simulink model "Ecm_2RC_battery"  (R2022a)
settings: Solver=FixedStepAuto  StartTime=0.0  StopTime=3600  FixedStep=0.1  RelTol=1e-3
values from neighbouring files (symbols this model uses):
  T_init = 293.15    [cell_data.mat]
libraries: fl_lib x1074, LiBatteryElements_lib x540, nesl_utility x102
(part 2 of 18)

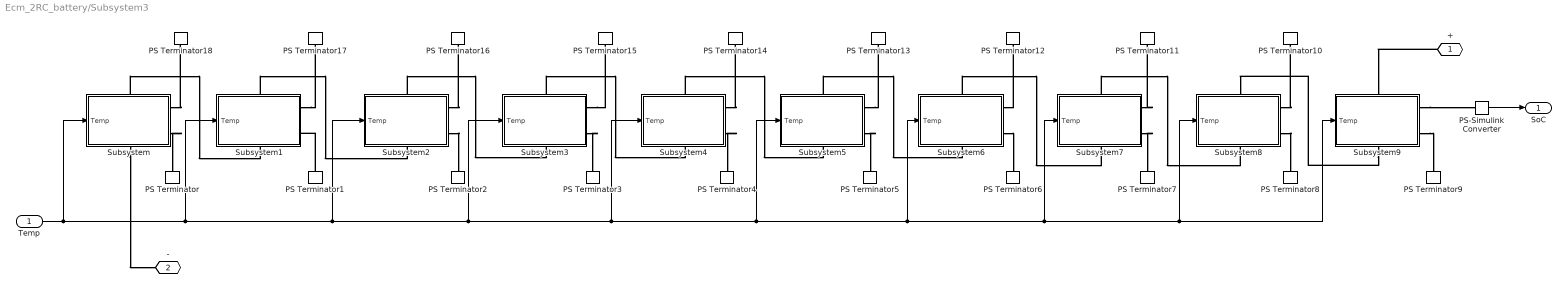
== system Ecm_2RC_battery/Subsystem3 ==
  Temp : Inport
  PS Terminator{,1..18} (19 alike) : fl_lib/Physical Signals/Sinks/PS Terminator
      settings: SourceProductBaseCode=PW,SS,VE
  PS-Simulink Converter : nesl_utility/PS-Simulink Converter  PhysicalDomain=network_engine_domain  SubClassName=ps_output  LeftPortType=input  RightPortType=output  PseudoPeriodic=off  Frequencies=[]  VectorFormat=inherit  Unit=inherit  AffineConversion=off
      settings: SourceProductBaseCode=SS,PW,VE
  Subsystem : Subsystem
      settings: PortSchema="{\"entries\":[{\"content\":{\"sides\":[{\"content\":{\"connectorIds\":[\"In1\"]},\"type\":\"ConnectorPlacement.EquallySpacedRectSide\",\"uuid\":\"c40d362d-5d22-4f8a-8be9-1546116d818f\"},{\"content\":{\"connectorIds\":[\"RConn1\",\"RConn2\"],\"side\":\"RIGHT\"},\"type\":\"ConnectorPlacement.EquallySpacedRectSide\",\"uuid\":\"b280b04f-a99a-4e6d-85c5-70766288d403\"},{\"content\":{\"connectorIds\":[\"LConn1\"],\"side\":\"TOP\"},\"type\":\"ConnectorPlacement.EquallySpacedRectSide\",\"uuid\":\"c08bcee5-d382-416b-973d-9a8915fb752a\"},{\"content\":{\"connectorIds\":[\"RConn3\"],\"side\":\"BOTTOM\"},\"type\":\"ConnectorPlacement.EquallySpacedRectSide\",\"uuid\":\"7b01a887-c5d2-42f0-ba08-9cc04bc53540\"}]},\"type\":\"ConnectorPlacement.EquallySpacedConnector\",\"uuid\":\"7a443456-32e2-4b79-b23a-7f1f6189d6a8\"}],\"packageUris\":[\"http://schema.mathworks.com/mf0/Connector/R2020b\"],\"version\":\"1.0\"}"
  Subsystem1 : Subsystem
      settings: PortSchema="{\"entries\":[{\"content\":{\"sides\":[{\"content\":{\"connectorIds\":[\"In1\"]},\"type\":\"ConnectorPlacement.EquallySpacedRectSide\",\"uuid\":\"c40d362d-5d22-4f8a-8be9-1546116d818f\"},{\"content\":{\"connectorIds\":[\"RConn1\",\"RConn2\"],\"side\":\"RIGHT\"},\"type\":\"ConnectorPlacement.EquallySpacedRectSide\",\"uuid\":\"b280b04f-a99a-4e6d-85c5-70766288d403\"},{\"content\":{\"connectorIds\":[\"LConn1\"],\"side\":\"TOP\"},\"type\":\"ConnectorPlacement.EquallySpacedRectSide\",\"uuid\":\"c08bcee5-d382-416b-973d-9a8915fb752a\"},{\"content\":{\"connectorIds\":[\"RConn3\"],\"side\":\"BOTTOM\"},\"type\":\"ConnectorPlacement.EquallySpacedRectSide\",\"uuid\":\"7b01a887-c5d2-42f0-ba08-9cc04bc53540\"}]},\"type\":\"ConnectorPlacement.EquallySpacedConnector\",\"uuid\":\"7a443456-32e2-4b79-b23a-7f1f6189d6a8\"}],\"packageUris\":[\"http://schema.mathworks.com/mf0/Connector/R2020b\"],\"version\":\"1.0\"}"
  Subsystem2 : Subsystem
      settings: PortSchema="{\"entries\":[{\"content\":{\"sides\":[{\"content\":{\"connectorIds\":[\"In1\"]},\"type\":\"ConnectorPlacement.EquallySpacedRectSide\",\"uuid\":\"c40d362d-5d22-4f8a-8be9-1546116d818f\"},{\"content\":{\"connectorIds\":[\"RConn1\",\"RConn2\"],\"side\":\"RIGHT\"},\"type\":\"ConnectorPlacement.EquallySpacedRectSide\",\"uuid\":\"b280b04f-a99a-4e6d-85c5-70766288d403\"},{\"content\":{\"connectorIds\":[\"LConn1\"],\"side\":\"TOP\"},\"type\":\"ConnectorPlacement.EquallySpacedRectSide\",\"uuid\":\"c08bcee5-d382-416b-973d-9a8915fb752a\"},{\"content\":{\"connectorIds\":[\"RConn3\"],\"side\":\"BOTTOM\"},\"type\":\"ConnectorPlacement.EquallySpacedRectSide\",\"uuid\":\"7b01a887-c5d2-42f0-ba08-9cc04bc53540\"}]},\"type\":\"ConnectorPlacement.EquallySpacedConnector\",\"uuid\":\"7a443456-32e2-4b79-b23a-7f1f6189d6a8\"}],\"packageUris\":[\"http://schema.mathworks.com/mf0/Connector/R2020b\"],\"version\":\"1.0\"}"
  Subsystem3 : Subsystem
      settings: PortSchema="{\"entries\":[{\"content\":{\"sides\":[{\"content\":{\"connectorIds\":[\"In1\"]},\"type\":\"ConnectorPlacement.EquallySpacedRectSide\",\"uuid\":\"c40d362d-5d22-4f8a-8be9-1546116d818f\"},{\"content\":{\"connectorIds\":[\"RConn1\",\"RConn2\"],\"side\":\"RIGHT\"},\"type\":\"ConnectorPlacement.EquallySpacedRectSide\",\"uuid\":\"b280b04f-a99a-4e6d-85c5-70766288d403\"},{\"content\":{\"connectorIds\":[\"LConn1\"],\"side\":\"TOP\"},\"type\":\"ConnectorPlacement.EquallySpacedRectSide\",\"uuid\":\"c08bcee5-d382-416b-973d-9a8915fb752a\"},{\"content\":{\"connectorIds\":[\"RConn3\"],\"side\":\"BOTTOM\"},\"type\":\"ConnectorPlacement.EquallySpacedRectSide\",\"uuid\":\"7b01a887-c5d2-42f0-ba08-9cc04bc53540\"}]},\"type\":\"ConnectorPlacement.EquallySpacedConnector\",\"uuid\":\"7a443456-32e2-4b79-b23a-7f1f6189d6a8\"}],\"packageUris\":[\"http://schema.mathworks.com/mf0/Connector/R2020b\"],\"version\":\"1.0\"}"
  Subsystem4 : Subsystem
      settings: PortSchema="{\"entries\":[{\"content\":{\"sides\":[{\"content\":{\"connectorIds\":[\"In1\"]},\"type\":\"ConnectorPlacement.EquallySpacedRectSide\",\"uuid\":\"c40d362d-5d22-4f8a-8be9-1546116d818f\"},{\"content\":{\"connectorIds\":[\"RConn1\",\"RConn2\"],\"side\":\"RIGHT\"},\"type\":\"ConnectorPlacement.EquallySpacedRectSide\",\"uuid\":\"b280b04f-a99a-4e6d-85c5-70766288d403\"},{\"content\":{\"connectorIds\":[\"LConn1\"],\"side\":\"TOP\"},\"type\":\"ConnectorPlacement.EquallySpacedRectSide\",\"uuid\":\"c08bcee5-d382-416b-973d-9a8915fb752a\"},{\"content\":{\"connectorIds\":[\"RConn3\"],\"side\":\"BOTTOM\"},\"type\":\"ConnectorPlacement.EquallySpacedRectSide\",\"uuid\":\"7b01a887-c5d2-42f0-ba08-9cc04bc53540\"}]},\"type\":\"ConnectorPlacement.EquallySpacedConnector\",\"uuid\":\"7a443456-32e2-4b79-b23a-7f1f6189d6a8\"}],\"packageUris\":[\"http://schema.mathworks.com/mf0/Connector/R2020b\"],\"version\":\"1.0\"}"
  Subsystem5 : Subsystem
      settings: PortSchema="{\"entries\":[{\"content\":{\"sides\":[{\"content\":{\"connectorIds\":[\"In1\"]},\"type\":\"ConnectorPlacement.EquallySpacedRectSide\",\"uuid\":\"c40d362d-5d22-4f8a-8be9-1546116d818f\"},{\"content\":{\"connectorIds\":[\"RConn1\",\"RConn2\"],\"side\":\"RIGHT\"},\"type\":\"ConnectorPlacement.EquallySpacedRectSide\",\"uuid\":\"b280b04f-a99a-4e6d-85c5-70766288d403\"},{\"content\":{\"connectorIds\":[\"LConn1\"],\"side\":\"TOP\"},\"type\":\"ConnectorPlacement.EquallySpacedRectSide\",\"uuid\":\"c08bcee5-d382-416b-973d-9a8915fb752a\"},{\"content\":{\"connectorIds\":[\"RConn3\"],\"side\":\"BOTTOM\"},\"type\":\"ConnectorPlacement.EquallySpacedRectSide\",\"uuid\":\"7b01a887-c5d2-42f0-ba08-9cc04bc53540\"}]},\"type\":\"ConnectorPlacement.EquallySpacedConnector\",\"uuid\":\"7a443456-32e2-4b79-b23a-7f1f6189d6a8\"}],\"packageUris\":[\"http://schema.mathworks.com/mf0/Connector/R2020b\"],\"version\":\"1.0\"}"
  Subsystem6 : Subsystem
      settings: PortSchema="{\"entries\":[{\"content\":{\"sides\":[{\"content\":{\"connectorIds\":[\"In1\"]},\"type\":\"ConnectorPlacement.EquallySpacedRectSide\",\"uuid\":\"c40d362d-5d22-4f8a-8be9-1546116d818f\"},{\"content\":{\"connectorIds\":[\"RConn1\",\"RConn2\"],\"side\":\"RIGHT\"},\"type\":\"ConnectorPlacement.EquallySpacedRectSide\",\"uuid\":\"b280b04f-a99a-4e6d-85c5-70766288d403\"},{\"content\":{\"connectorIds\":[\"LConn1\"],\"side\":\"TOP\"},\"type\":\"ConnectorPlacement.EquallySpacedRectSide\",\"uuid\":\"c08bcee5-d382-416b-973d-9a8915fb752a\"},{\"content\":{\"connectorIds\":[\"RConn3\"],\"side\":\"BOTTOM\"},\"type\":\"ConnectorPlacement.EquallySpacedRectSide\",\"uuid\":\"7b01a887-c5d2-42f0-ba08-9cc04bc53540\"}]},\"type\":\"ConnectorPlacement.EquallySpacedConnector\",\"uuid\":\"7a443456-32e2-4b79-b23a-7f1f6189d6a8\"}],\"packageUris\":[\"http://schema.mathworks.com/mf0/Connector/R2020b\"],\"version\":\"1.0\"}"
  Subsystem7 : Subsystem
      settings: PortSchema="{\"entries\":[{\"content\":{\"sides\":[{\"content\":{\"connectorIds\":[\"In1\"]},\"type\":\"ConnectorPlacement.EquallySpacedRectSide\",\"uuid\":\"c40d362d-5d22-4f8a-8be9-1546116d818f\"},{\"content\":{\"connectorIds\":[\"RConn1\",\"RConn2\"],\"side\":\"RIGHT\"},\"type\":\"ConnectorPlacement.EquallySpacedRectSide\",\"uuid\":\"b280b04f-a99a-4e6d-85c5-70766288d403\"},{\"content\":{\"connectorIds\":[\"LConn1\"],\"side\":\"TOP\"},\"type\":\"ConnectorPlacement.EquallySpacedRectSide\",\"uuid\":\"c08bcee5-d382-416b-973d-9a8915fb752a\"},{\"content\":{\"connectorIds\":[\"RConn3\"],\"side\":\"BOTTOM\"},\"type\":\"ConnectorPlacement.EquallySpacedRectSide\",\"uuid\":\"7b01a887-c5d2-42f0-ba08-9cc04bc53540\"}]},\"type\":\"ConnectorPlacement.EquallySpacedConnector\",\"uuid\":\"7a443456-32e2-4b79-b23a-7f1f6189d6a8\"}],\"packageUris\":[\"http://schema.mathworks.com/mf0/Connector/R2020b\"],\"version\":\"1.0\"}"
  Subsystem8 : Subsystem
      settings: PortSchema="{\"entries\":[{\"content\":{\"sides\":[{\"content\":{\"connectorIds\":[\"In1\"]},\"type\":\"ConnectorPlacement.EquallySpacedRectSide\",\"uuid\":\"c40d362d-5d22-4f8a-8be9-1546116d818f\"},{\"content\":{\"connectorIds\":[\"RConn1\",\"RConn2\"],\"side\":\"RIGHT\"},\"type\":\"ConnectorPlacement.EquallySpacedRectSide\",\"uuid\":\"b280b04f-a99a-4e6d-85c5-70766288d403\"},{\"content\":{\"connectorIds\":[\"LConn1\"],\"side\":\"TOP\"},\"type\":\"ConnectorPlacement.EquallySpacedRectSide\",\"uuid\":\"c08bcee5-d382-416b-973d-9a8915fb752a\"},{\"content\":{\"connectorIds\":[\"RConn3\"],\"side\":\"BOTTOM\"},\"type\":\"ConnectorPlacement.EquallySpacedRectSide\",\"uuid\":\"7b01a887-c5d2-42f0-ba08-9cc04bc53540\"}]},\"type\":\"ConnectorPlacement.EquallySpacedConnector\",\"uuid\":\"7a443456-32e2-4b79-b23a-7f1f6189d6a8\"}],\"packageUris\":[\"http://schema.mathworks.com/mf0/Connector/R2020b\"],\"version\":\"1.0\"}"
  Subsystem9 : Subsystem
      settings: PortSchema="{\"entries\":[{\"content\":{\"sides\":[{\"content\":{\"connectorIds\":[\"In1\"]},\"type\":\"ConnectorPlacement.EquallySpacedRectSide\",\"uuid\":\"c40d362d-5d22-4f8a-8be9-1546116d818f\"},{\"content\":{\"connectorIds\":[\"RConn1\",\"RConn2\"],\"side\":\"RIGHT\"},\"type\":\"ConnectorPlacement.EquallySpacedRectSide\",\"uuid\":\"b280b04f-a99a-4e6d-85c5-70766288d403\"},{\"content\":{\"connectorIds\":[\"LConn1\"],\"side\":\"TOP\"},\"type\":\"ConnectorPlacement.EquallySpacedRectSide\",\"uuid\":\"c08bcee5-d382-416b-973d-9a8915fb752a\"},{\"content\":{\"connectorIds\":[\"RConn3\"],\"side\":\"BOTTOM\"},\"type\":\"ConnectorPlacement.EquallySpacedRectSide\",\"uuid\":\"7b01a887-c5d2-42f0-ba08-9cc04bc53540\"}]},\"type\":\"ConnectorPlacement.EquallySpacedConnector\",\"uuid\":\"7a443456-32e2-4b79-b23a-7f1f6189d6a8\"}],\"packageUris\":[\"http://schema.mathworks.com/mf0/Connector/R2020b\"],\"version\":\"1.0\"}"
  + : PMIOPort  Side=Left
  - : PMIOPort  Port=2  Side=Right
  SoC : Outport
  wires:
  Temp/1 -> Subsystem1/1(Temp), Subsystem2/1(Temp), Subsystem3/1(Temp), Subsystem4/1(Temp), Subsystem7/1(Temp), Subsystem9/1(Temp), Subsystem8/1(Temp), Subsystem6/1(Temp), Subsystem5/1(Temp), Subsystem/1(Temp)
  PS-Simulink Converter/1 -> SoC/1
  connections:
  Subsystem7/RConn1 -- PS Terminator11/LConn1
  Subsystem1/RConn1 -- PS Terminator17/LConn1
  Subsystem5/RConn2 -- PS Terminator5/LConn1
  Subsystem4/RConn1 -- PS Terminator14/LConn1
  Subsystem8/RConn2 -- PS Terminator8/LConn1
  Subsystem4/RConn2 -- PS Terminator4/LConn1
  Subsystem9/RConn1 -- PS-Simulink Converter/LConn1
  Subsystem5/RConn1 -- PS Terminator13/LConn1
  Subsystem6/RConn1 -- PS Terminator12/LConn1
  Subsystem/RConn1 -- PS Terminator18/LConn1
  Subsystem3/RConn2 -- PS Terminator3/LConn1
  Subsystem5/LConn1 -- Subsystem6/RConn3
  +/RConn1 -- Subsystem9/LConn1
  Subsystem6/RConn2 -- PS Terminator6/LConn1
  Subsystem2/RConn2 -- PS Terminator2/LConn1
  Subsystem9/RConn3 -- Subsystem8/LConn1
  Subsystem2/LConn1 -- Subsystem3/RConn3
  Subsystem/RConn2 -- PS Terminator/LConn1
  Subsystem7/LConn1 -- Subsystem8/RConn3
  Subsystem9/RConn2 -- PS Terminator9/LConn1
  Subsystem7/RConn2 -- PS Terminator7/LConn1
  Subsystem/LConn1 -- Subsystem1/RConn3
  Subsystem1/LConn1 -- Subsystem2/RConn3
  Subsystem/RConn3 -- -/RConn1
  Subsystem4/LConn1 -- Subsystem5/RConn3
  Subsystem6/LConn1 -- Subsystem7/RConn3
  Subsystem2/RConn1 -- PS Terminator16/LConn1
  Subsystem3/LConn1 -- Subsystem4/RConn3
  Subsystem3/RConn1 -- PS Terminator15/LConn1
  PS Terminator1/LConn1 -- Subsystem1/RConn2
  Subsystem8/RConn1 -- PS Terminator10/LConn1

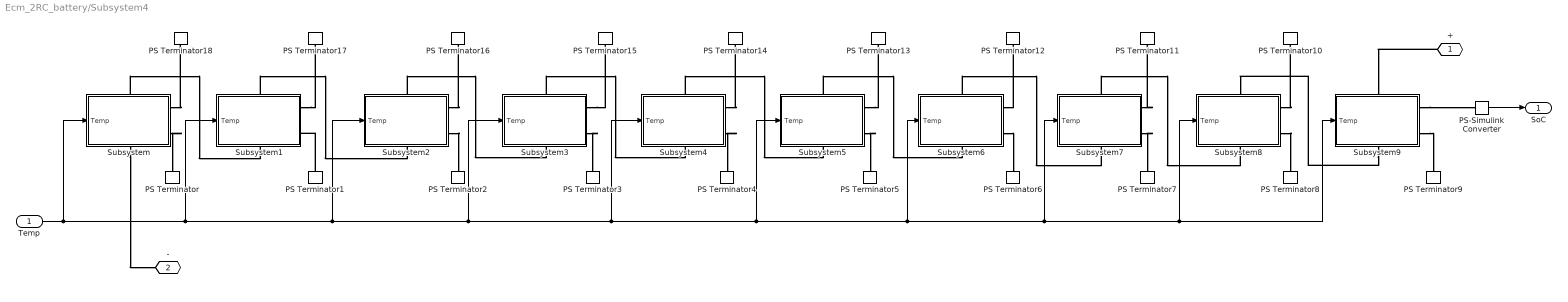
== system Ecm_2RC_battery/Subsystem4 ==
  Temp : Inport
  PS Terminator{,1..18} (19 alike) : fl_lib/Physical Signals/Sinks/PS Terminator
      settings: SourceProductBaseCode=PW,SS,VE
  PS-Simulink Converter : nesl_utility/PS-Simulink Converter  PhysicalDomain=network_engine_domain  SubClassName=ps_output  LeftPortType=input  RightPortType=output  PseudoPeriodic=off  Frequencies=[]  VectorFormat=inherit  Unit=inherit  AffineConversion=off
      settings: SourceProductBaseCode=SS,PW,VE
  Subsystem : Subsystem
      settings: PortSchema="{\"entries\":[{\"content\":{\"sides\":[{\"content\":{\"connectorIds\":[\"In1\"]},\"type\":\"ConnectorPlacement.EquallySpacedRectSide\",\"uuid\":\"c40d362d-5d22-4f8a-8be9-1546116d818f\"},{\"content\":{\"connectorIds\":[\"RConn1\",\"RConn2\"],\"side\":\"RIGHT\"},\"type\":\"ConnectorPlacement.EquallySpacedRectSide\",\"uuid\":\"b280b04f-a99a-4e6d-85c5-70766288d403\"},{\"content\":{\"connectorIds\":[\"LConn1\"],\"side\":\"TOP\"},\"type\":\"ConnectorPlacement.EquallySpacedRectSide\",\"uuid\":\"c08bcee5-d382-416b-973d-9a8915fb752a\"},{\"content\":{\"connectorIds\":[\"RConn3\"],\"side\":\"BOTTOM\"},\"type\":\"ConnectorPlacement.EquallySpacedRectSide\",\"uuid\":\"7b01a887-c5d2-42f0-ba08-9cc04bc53540\"}]},\"type\":\"ConnectorPlacement.EquallySpacedConnector\",\"uuid\":\"7a443456-32e2-4b79-b23a-7f1f6189d6a8\"}],\"packageUris\":[\"http://schema.mathworks.com/mf0/Connector/R2020b\"],\"version\":\"1.0\"}"
  Subsystem1 : Subsystem
      settings: PortSchema="{\"entries\":[{\"content\":{\"sides\":[{\"content\":{\"connectorIds\":[\"In1\"]},\"type\":\"ConnectorPlacement.EquallySpacedRectSide\",\"uuid\":\"c40d362d-5d22-4f8a-8be9-1546116d818f\"},{\"content\":{\"connectorIds\":[\"RConn1\",\"RConn2\"],\"side\":\"RIGHT\"},\"type\":\"ConnectorPlacement.EquallySpacedRectSide\",\"uuid\":\"b280b04f-a99a-4e6d-85c5-70766288d403\"},{\"content\":{\"connectorIds\":[\"LConn1\"],\"side\":\"TOP\"},\"type\":\"ConnectorPlacement.EquallySpacedRectSide\",\"uuid\":\"c08bcee5-d382-416b-973d-9a8915fb752a\"},{\"content\":{\"connectorIds\":[\"RConn3\"],\"side\":\"BOTTOM\"},\"type\":\"ConnectorPlacement.EquallySpacedRectSide\",\"uuid\":\"7b01a887-c5d2-42f0-ba08-9cc04bc53540\"}]},\"type\":\"ConnectorPlacement.EquallySpacedConnector\",\"uuid\":\"7a443456-32e2-4b79-b23a-7f1f6189d6a8\"}],\"packageUris\":[\"http://schema.mathworks.com/mf0/Connector/R2020b\"],\"version\":\"1.0\"}"
  Subsystem2 : Subsystem
      settings: PortSchema="{\"entries\":[{\"content\":{\"sides\":[{\"content\":{\"connectorIds\":[\"In1\"]},\"type\":\"ConnectorPlacement.EquallySpacedRectSide\",\"uuid\":\"c40d362d-5d22-4f8a-8be9-1546116d818f\"},{\"content\":{\"connectorIds\":[\"RConn1\",\"RConn2\"],\"side\":\"RIGHT\"},\"type\":\"ConnectorPlacement.EquallySpacedRectSide\",\"uuid\":\"b280b04f-a99a-4e6d-85c5-70766288d403\"},{\"content\":{\"connectorIds\":[\"LConn1\"],\"side\":\"TOP\"},\"type\":\"ConnectorPlacement.EquallySpacedRectSide\",\"uuid\":\"c08bcee5-d382-416b-973d-9a8915fb752a\"},{\"content\":{\"connectorIds\":[\"RConn3\"],\"side\":\"BOTTOM\"},\"type\":\"ConnectorPlacement.EquallySpacedRectSide\",\"uuid\":\"7b01a887-c5d2-42f0-ba08-9cc04bc53540\"}]},\"type\":\"ConnectorPlacement.EquallySpacedConnector\",\"uuid\":\"7a443456-32e2-4b79-b23a-7f1f6189d6a8\"}],\"packageUris\":[\"http://schema.mathworks.com/mf0/Connector/R2020b\"],\"version\":\"1.0\"}"
  Subsystem3 : Subsystem
      settings: PortSchema="{\"entries\":[{\"content\":{\"sides\":[{\"content\":{\"connectorIds\":[\"In1\"]},\"type\":\"ConnectorPlacement.EquallySpacedRectSide\",\"uuid\":\"c40d362d-5d22-4f8a-8be9-1546116d818f\"},{\"content\":{\"connectorIds\":[\"RConn1\",\"RConn2\"],\"side\":\"RIGHT\"},\"type\":\"ConnectorPlacement.EquallySpacedRectSide\",\"uuid\":\"b280b04f-a99a-4e6d-85c5-70766288d403\"},{\"content\":{\"connectorIds\":[\"LConn1\"],\"side\":\"TOP\"},\"type\":\"ConnectorPlacement.EquallySpacedRectSide\",\"uuid\":\"c08bcee5-d382-416b-973d-9a8915fb752a\"},{\"content\":{\"connectorIds\":[\"RConn3\"],\"side\":\"BOTTOM\"},\"type\":\"ConnectorPlacement.EquallySpacedRectSide\",\"uuid\":\"7b01a887-c5d2-42f0-ba08-9cc04bc53540\"}]},\"type\":\"ConnectorPlacement.EquallySpacedConnector\",\"uuid\":\"7a443456-32e2-4b79-b23a-7f1f6189d6a8\"}],\"packageUris\":[\"http://schema.mathworks.com/mf0/Connector/R2020b\"],\"version\":\"1.0\"}"
  Subsystem4 : Subsystem
      settings: PortSchema="{\"entries\":[{\"content\":{\"sides\":[{\"content\":{\"connectorIds\":[\"In1\"]},\"type\":\"ConnectorPlacement.EquallySpacedRectSide\",\"uuid\":\"c40d362d-5d22-4f8a-8be9-1546116d818f\"},{\"content\":{\"connectorIds\":[\"RConn1\",\"RConn2\"],\"side\":\"RIGHT\"},\"type\":\"ConnectorPlacement.EquallySpacedRectSide\",\"uuid\":\"b280b04f-a99a-4e6d-85c5-70766288d403\"},{\"content\":{\"connectorIds\":[\"LConn1\"],\"side\":\"TOP\"},\"type\":\"ConnectorPlacement.EquallySpacedRectSide\",\"uuid\":\"c08bcee5-d382-416b-973d-9a8915fb752a\"},{\"content\":{\"connectorIds\":[\"RConn3\"],\"side\":\"BOTTOM\"},\"type\":\"ConnectorPlacement.EquallySpacedRectSide\",\"uuid\":\"7b01a887-c5d2-42f0-ba08-9cc04bc53540\"}]},\"type\":\"ConnectorPlacement.EquallySpacedConnector\",\"uuid\":\"7a443456-32e2-4b79-b23a-7f1f6189d6a8\"}],\"packageUris\":[\"http://schema.mathworks.com/mf0/Connector/R2020b\"],\"version\":\"1.0\"}"
  Subsystem5 : Subsystem
      settings: PortSchema="{\"entries\":[{\"content\":{\"sides\":[{\"content\":{\"connectorIds\":[\"In1\"]},\"type\":\"ConnectorPlacement.EquallySpacedRectSide\",\"uuid\":\"c40d362d-5d22-4f8a-8be9-1546116d818f\"},{\"content\":{\"connectorIds\":[\"RConn1\",\"RConn2\"],\"side\":\"RIGHT\"},\"type\":\"ConnectorPlacement.EquallySpacedRectSide\",\"uuid\":\"b280b04f-a99a-4e6d-85c5-70766288d403\"},{\"content\":{\"connectorIds\":[\"LConn1\"],\"side\":\"TOP\"},\"type\":\"ConnectorPlacement.EquallySpacedRectSide\",\"uuid\":\"c08bcee5-d382-416b-973d-9a8915fb752a\"},{\"content\":{\"connectorIds\":[\"RConn3\"],\"side\":\"BOTTOM\"},\"type\":\"ConnectorPlacement.EquallySpacedRectSide\",\"uuid\":\"7b01a887-c5d2-42f0-ba08-9cc04bc53540\"}]},\"type\":\"ConnectorPlacement.EquallySpacedConnector\",\"uuid\":\"7a443456-32e2-4b79-b23a-7f1f6189d6a8\"}],\"packageUris\":[\"http://schema.mathworks.com/mf0/Connector/R2020b\"],\"version\":\"1.0\"}"
  Subsystem6 : Subsystem
      settings: PortSchema="{\"entries\":[{\"content\":{\"sides\":[{\"content\":{\"connectorIds\":[\"In1\"]},\"type\":\"ConnectorPlacement.EquallySpacedRectSide\",\"uuid\":\"c40d362d-5d22-4f8a-8be9-1546116d818f\"},{\"content\":{\"connectorIds\":[\"RConn1\",\"RConn2\"],\"side\":\"RIGHT\"},\"type\":\"ConnectorPlacement.EquallySpacedRectSide\",\"uuid\":\"b280b04f-a99a-4e6d-85c5-70766288d403\"},{\"content\":{\"connectorIds\":[\"LConn1\"],\"side\":\"TOP\"},\"type\":\"ConnectorPlacement.EquallySpacedRectSide\",\"uuid\":\"c08bcee5-d382-416b-973d-9a8915fb752a\"},{\"content\":{\"connectorIds\":[\"RConn3\"],\"side\":\"BOTTOM\"},\"type\":\"ConnectorPlacement.EquallySpacedRectSide\",\"uuid\":\"7b01a887-c5d2-42f0-ba08-9cc04bc53540\"}]},\"type\":\"ConnectorPlacement.EquallySpacedConnector\",\"uuid\":\"7a443456-32e2-4b79-b23a-7f1f6189d6a8\"}],\"packageUris\":[\"http://schema.mathworks.com/mf0/Connector/R2020b\"],\"version\":\"1.0\"}"
  Subsystem7 : Subsystem
      settings: PortSchema="{\"entries\":[{\"content\":{\"sides\":[{\"content\":{\"connectorIds\":[\"In1\"]},\"type\":\"ConnectorPlacement.EquallySpacedRectSide\",\"uuid\":\"c40d362d-5d22-4f8a-8be9-1546116d818f\"},{\"content\":{\"connectorIds\":[\"RConn1\",\"RConn2\"],\"side\":\"RIGHT\"},\"type\":\"ConnectorPlacement.EquallySpacedRectSide\",\"uuid\":\"b280b04f-a99a-4e6d-85c5-70766288d403\"},{\"content\":{\"connectorIds\":[\"LConn1\"],\"side\":\"TOP\"},\"type\":\"ConnectorPlacement.EquallySpacedRectSide\",\"uuid\":\"c08bcee5-d382-416b-973d-9a8915fb752a\"},{\"content\":{\"connectorIds\":[\"RConn3\"],\"side\":\"BOTTOM\"},\"type\":\"ConnectorPlacement.EquallySpacedRectSide\",\"uuid\":\"7b01a887-c5d2-42f0-ba08-9cc04bc53540\"}]},\"type\":\"ConnectorPlacement.EquallySpacedConnector\",\"uuid\":\"7a443456-32e2-4b79-b23a-7f1f6189d6a8\"}],\"packageUris\":[\"http://schema.mathworks.com/mf0/Connector/R2020b\"],\"version\":\"1.0\"}"
  Subsystem8 : Subsystem
      settings: PortSchema="{\"entries\":[{\"content\":{\"sides\":[{\"content\":{\"connectorIds\":[\"In1\"]},\"type\":\"ConnectorPlacement.EquallySpacedRectSide\",\"uuid\":\"c40d362d-5d22-4f8a-8be9-1546116d818f\"},{\"content\":{\"connectorIds\":[\"RConn1\",\"RConn2\"],\"side\":\"RIGHT\"},\"type\":\"ConnectorPlacement.EquallySpacedRectSide\",\"uuid\":\"b280b04f-a99a-4e6d-85c5-70766288d403\"},{\"content\":{\"connectorIds\":[\"LConn1\"],\"side\":\"TOP\"},\"type\":\"ConnectorPlacement.EquallySpacedRectSide\",\"uuid\":\"c08bcee5-d382-416b-973d-9a8915fb752a\"},{\"content\":{\"connectorIds\":[\"RConn3\"],\"side\":\"BOTTOM\"},\"type\":\"ConnectorPlacement.EquallySpacedRectSide\",\"uuid\":\"7b01a887-c5d2-42f0-ba08-9cc04bc53540\"}]},\"type\":\"ConnectorPlacement.EquallySpacedConnector\",\"uuid\":\"7a443456-32e2-4b79-b23a-7f1f6189d6a8\"}],\"packageUris\":[\"http://schema.mathworks.com/mf0/Connector/R2020b\"],\"version\":\"1.0\"}"
  Subsystem9 : Subsystem
      settings: PortSchema="{\"entries\":[{\"content\":{\"sides\":[{\"content\":{\"connectorIds\":[\"In1\"]},\"type\":\"ConnectorPlacement.EquallySpacedRectSide\",\"uuid\":\"c40d362d-5d22-4f8a-8be9-1546116d818f\"},{\"content\":{\"connectorIds\":[\"RConn1\",\"RConn2\"],\"side\":\"RIGHT\"},\"type\":\"ConnectorPlacement.EquallySpacedRectSide\",\"uuid\":\"b280b04f-a99a-4e6d-85c5-70766288d403\"},{\"content\":{\"connectorIds\":[\"LConn1\"],\"side\":\"TOP\"},\"type\":\"ConnectorPlacement.EquallySpacedRectSide\",\"uuid\":\"c08bcee5-d382-416b-973d-9a8915fb752a\"},{\"content\":{\"connectorIds\":[\"RConn3\"],\"side\":\"BOTTOM\"},\"type\":\"ConnectorPlacement.EquallySpacedRectSide\",\"uuid\":\"7b01a887-c5d2-42f0-ba08-9cc04bc53540\"}]},\"type\":\"ConnectorPlacement.EquallySpacedConnector\",\"uuid\":\"7a443456-32e2-4b79-b23a-7f1f6189d6a8\"}],\"packageUris\":[\"http://schema.mathworks.com/mf0/Connector/R2020b\"],\"version\":\"1.0\"}"
  + : PMIOPort  Side=Left
  - : PMIOPort  Port=2  Side=Right
  SoC : Outport
  wires:
  Temp/1 -> Subsystem1/1(Temp), Subsystem2/1(Temp), Subsystem3/1(Temp), Subsystem4/1(Temp), Subsystem7/1(Temp), Subsystem9/1(Temp), Subsystem8/1(Temp), Subsystem6/1(Temp), Subsystem5/1(Temp), Subsystem/1(Temp)
  PS-Simulink Converter/1 -> SoC/1
  connections:
  Subsystem7/RConn1 -- PS Terminator11/LConn1
  Subsystem1/RConn1 -- PS Terminator17/LConn1
  Subsystem5/RConn2 -- PS Terminator5/LConn1
  Subsystem4/RConn1 -- PS Terminator14/LConn1
  Subsystem8/RConn2 -- PS Terminator8/LConn1
  Subsystem4/RConn2 -- PS Terminator4/LConn1
  Subsystem9/RConn1 -- PS-Simulink Converter/LConn1
  Subsystem5/RConn1 -- PS Terminator13/LConn1
  Subsystem6/RConn1 -- PS Terminator12/LConn1
  Subsystem/RConn1 -- PS Terminator18/LConn1
  Subsystem3/RConn2 -- PS Terminator3/LConn1
  Subsystem5/LConn1 -- Subsystem6/RConn3
  +/RConn1 -- Subsystem9/LConn1
  Subsystem6/RConn2 -- PS Terminator6/LConn1
  Subsystem2/RConn2 -- PS Terminator2/LConn1
  Subsystem9/RConn3 -- Subsystem8/LConn1
  Subsystem2/LConn1 -- Subsystem3/RConn3
  Subsystem/RConn2 -- PS Terminator/LConn1
  Subsystem7/LConn1 -- Subsystem8/RConn3
  Subsystem9/RConn2 -- PS Terminator9/LConn1
  Subsystem7/RConn2 -- PS Terminator7/LConn1
  Subsystem/LConn1 -- Subsystem1/RConn3
  Subsystem1/LConn1 -- Subsystem2/RConn3
  Subsystem/RConn3 -- -/RConn1
  Subsystem4/LConn1 -- Subsystem5/RConn3
  Subsystem6/LConn1 -- Subsystem7/RConn3
  Subsystem2/RConn1 -- PS Terminator16/LConn1
  Subsystem3/LConn1 -- Subsystem4/RConn3
  Subsystem3/RConn1 -- PS Terminator15/LConn1
  PS Terminator1/LConn1 -- Subsystem1/RConn2
  Subsystem8/RConn1 -- PS Terminator10/LConn1

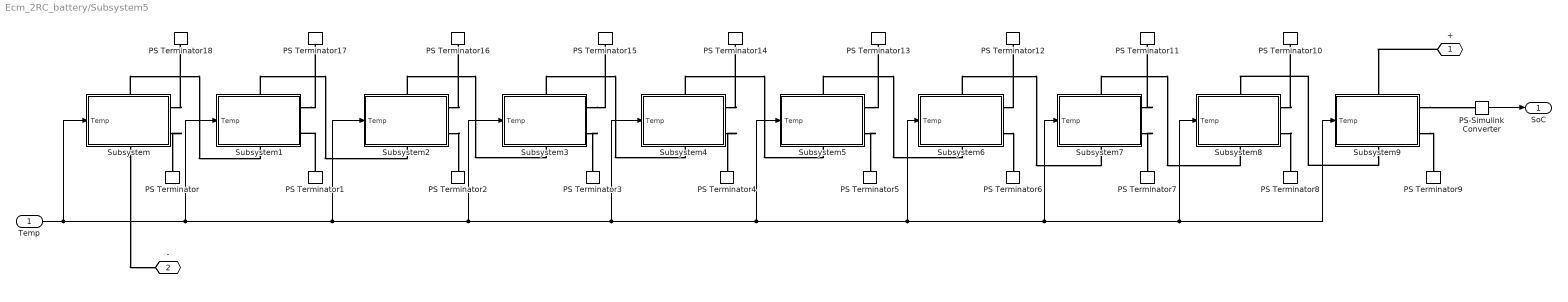
== system Ecm_2RC_battery/Subsystem5 ==
  Temp : Inport
  PS Terminator{,1..18} (19 alike) : fl_lib/Physical Signals/Sinks/PS Terminator
      settings: SourceProductBaseCode=PW,SS,VE
  PS-Simulink Converter : nesl_utility/PS-Simulink Converter  PhysicalDomain=network_engine_domain  SubClassName=ps_output  LeftPortType=input  RightPortType=output  PseudoPeriodic=off  Frequencies=[]  VectorFormat=inherit  Unit=inherit  AffineConversion=off
      settings: SourceProductBaseCode=SS,PW,VE
  Subsystem : Subsystem
      settings: PortSchema="{\"entries\":[{\"content\":{\"sides\":[{\"content\":{\"connectorIds\":[\"In1\"]},\"type\":\"ConnectorPlacement.EquallySpacedRectSide\",\"uuid\":\"c40d362d-5d22-4f8a-8be9-1546116d818f\"},{\"content\":{\"connectorIds\":[\"RConn1\",\"RConn2\"],\"side\":\"RIGHT\"},\"type\":\"ConnectorPlacement.EquallySpacedRectSide\",\"uuid\":\"b280b04f-a99a-4e6d-85c5-70766288d403\"},{\"content\":{\"connectorIds\":[\"LConn1\"],\"side\":\"TOP\"},\"type\":\"ConnectorPlacement.EquallySpacedRectSide\",\"uuid\":\"c08bcee5-d382-416b-973d-9a8915fb752a\"},{\"content\":{\"connectorIds\":[\"RConn3\"],\"side\":\"BOTTOM\"},\"type\":\"ConnectorPlacement.EquallySpacedRectSide\",\"uuid\":\"7b01a887-c5d2-42f0-ba08-9cc04bc53540\"}]},\"type\":\"ConnectorPlacement.EquallySpacedConnector\",\"uuid\":\"7a443456-32e2-4b79-b23a-7f1f6189d6a8\"}],\"packageUris\":[\"http://schema.mathworks.com/mf0/Connector/R2020b\"],\"version\":\"1.0\"}"
  Subsystem1 : Subsystem
      settings: PortSchema="{\"entries\":[{\"content\":{\"sides\":[{\"content\":{\"connectorIds\":[\"In1\"]},\"type\":\"ConnectorPlacement.EquallySpacedRectSide\",\"uuid\":\"c40d362d-5d22-4f8a-8be9-1546116d818f\"},{\"content\":{\"connectorIds\":[\"RConn1\",\"RConn2\"],\"side\":\"RIGHT\"},\"type\":\"ConnectorPlacement.EquallySpacedRectSide\",\"uuid\":\"b280b04f-a99a-4e6d-85c5-70766288d403\"},{\"content\":{\"connectorIds\":[\"LConn1\"],\"side\":\"TOP\"},\"type\":\"ConnectorPlacement.EquallySpacedRectSide\",\"uuid\":\"c08bcee5-d382-416b-973d-9a8915fb752a\"},{\"content\":{\"connectorIds\":[\"RConn3\"],\"side\":\"BOTTOM\"},\"type\":\"ConnectorPlacement.EquallySpacedRectSide\",\"uuid\":\"7b01a887-c5d2-42f0-ba08-9cc04bc53540\"}]},\"type\":\"ConnectorPlacement.EquallySpacedConnector\",\"uuid\":\"7a443456-32e2-4b79-b23a-7f1f6189d6a8\"}],\"packageUris\":[\"http://schema.mathworks.com/mf0/Connector/R2020b\"],\"version\":\"1.0\"}"
  Subsystem2 : Subsystem
      settings: PortSchema="{\"entries\":[{\"content\":{\"sides\":[{\"content\":{\"connectorIds\":[\"In1\"]},\"type\":\"ConnectorPlacement.EquallySpacedRectSide\",\"uuid\":\"c40d362d-5d22-4f8a-8be9-1546116d818f\"},{\"content\":{\"connectorIds\":[\"RConn1\",\"RConn2\"],\"side\":\"RIGHT\"},\"type\":\"ConnectorPlacement.EquallySpacedRectSide\",\"uuid\":\"b280b04f-a99a-4e6d-85c5-70766288d403\"},{\"content\":{\"connectorIds\":[\"LConn1\"],\"side\":\"TOP\"},\"type\":\"ConnectorPlacement.EquallySpacedRectSide\",\"uuid\":\"c08bcee5-d382-416b-973d-9a8915fb752a\"},{\"content\":{\"connectorIds\":[\"RConn3\"],\"side\":\"BOTTOM\"},\"type\":\"ConnectorPlacement.EquallySpacedRectSide\",\"uuid\":\"7b01a887-c5d2-42f0-ba08-9cc04bc53540\"}]},\"type\":\"ConnectorPlacement.EquallySpacedConnector\",\"uuid\":\"7a443456-32e2-4b79-b23a-7f1f6189d6a8\"}],\"packageUris\":[\"http://schema.mathworks.com/mf0/Connector/R2020b\"],\"version\":\"1.0\"}"
  Subsystem3 : Subsystem
      settings: PortSchema="{\"entries\":[{\"content\":{\"sides\":[{\"content\":{\"connectorIds\":[\"In1\"]},\"type\":\"ConnectorPlacement.EquallySpacedRectSide\",\"uuid\":\"c40d362d-5d22-4f8a-8be9-1546116d818f\"},{\"content\":{\"connectorIds\":[\"RConn1\",\"RConn2\"],\"side\":\"RIGHT\"},\"type\":\"ConnectorPlacement.EquallySpacedRectSide\",\"uuid\":\"b280b04f-a99a-4e6d-85c5-70766288d403\"},{\"content\":{\"connectorIds\":[\"LConn1\"],\"side\":\"TOP\"},\"type\":\"ConnectorPlacement.EquallySpacedRectSide\",\"uuid\":\"c08bcee5-d382-416b-973d-9a8915fb752a\"},{\"content\":{\"connectorIds\":[\"RConn3\"],\"side\":\"BOTTOM\"},\"type\":\"ConnectorPlacement.EquallySpacedRectSide\",\"uuid\":\"7b01a887-c5d2-42f0-ba08-9cc04bc53540\"}]},\"type\":\"ConnectorPlacement.EquallySpacedConnector\",\"uuid\":\"7a443456-32e2-4b79-b23a-7f1f6189d6a8\"}],\"packageUris\":[\"http://schema.mathworks.com/mf0/Connector/R2020b\"],\"version\":\"1.0\"}"
  Subsystem4 : Subsystem
      settings: PortSchema="{\"entries\":[{\"content\":{\"sides\":[{\"content\":{\"connectorIds\":[\"In1\"]},\"type\":\"ConnectorPlacement.EquallySpacedRectSide\",\"uuid\":\"c40d362d-5d22-4f8a-8be9-1546116d818f\"},{\"content\":{\"connectorIds\":[\"RConn1\",\"RConn2\"],\"side\":\"RIGHT\"},\"type\":\"ConnectorPlacement.EquallySpacedRectSide\",\"uuid\":\"b280b04f-a99a-4e6d-85c5-70766288d403\"},{\"content\":{\"connectorIds\":[\"LConn1\"],\"side\":\"TOP\"},\"type\":\"ConnectorPlacement.EquallySpacedRectSide\",\"uuid\":\"c08bcee5-d382-416b-973d-9a8915fb752a\"},{\"content\":{\"connectorIds\":[\"RConn3\"],\"side\":\"BOTTOM\"},\"type\":\"ConnectorPlacement.EquallySpacedRectSide\",\"uuid\":\"7b01a887-c5d2-42f0-ba08-9cc04bc53540\"}]},\"type\":\"ConnectorPlacement.EquallySpacedConnector\",\"uuid\":\"7a443456-32e2-4b79-b23a-7f1f6189d6a8\"}],\"packageUris\":[\"http://schema.mathworks.com/mf0/Connector/R2020b\"],\"version\":\"1.0\"}"
  Subsystem5 : Subsystem
      settings: PortSchema="{\"entries\":[{\"content\":{\"sides\":[{\"content\":{\"connectorIds\":[\"In1\"]},\"type\":\"ConnectorPlacement.EquallySpacedRectSide\",\"uuid\":\"c40d362d-5d22-4f8a-8be9-1546116d818f\"},{\"content\":{\"connectorIds\":[\"RConn1\",\"RConn2\"],\"side\":\"RIGHT\"},\"type\":\"ConnectorPlacement.EquallySpacedRectSide\",\"uuid\":\"b280b04f-a99a-4e6d-85c5-70766288d403\"},{\"content\":{\"connectorIds\":[\"LConn1\"],\"side\":\"TOP\"},\"type\":\"ConnectorPlacement.EquallySpacedRectSide\",\"uuid\":\"c08bcee5-d382-416b-973d-9a8915fb752a\"},{\"content\":{\"connectorIds\":[\"RConn3\"],\"side\":\"BOTTOM\"},\"type\":\"ConnectorPlacement.EquallySpacedRectSide\",\"uuid\":\"7b01a887-c5d2-42f0-ba08-9cc04bc53540\"}]},\"type\":\"ConnectorPlacement.EquallySpacedConnector\",\"uuid\":\"7a443456-32e2-4b79-b23a-7f1f6189d6a8\"}],\"packageUris\":[\"http://schema.mathworks.com/mf0/Connector/R2020b\"],\"version\":\"1.0\"}"
  Subsystem6 : Subsystem
      settings: PortSchema="{\"entries\":[{\"content\":{\"sides\":[{\"content\":{\"connectorIds\":[\"In1\"]},\"type\":\"ConnectorPlacement.EquallySpacedRectSide\",\"uuid\":\"c40d362d-5d22-4f8a-8be9-1546116d818f\"},{\"content\":{\"connectorIds\":[\"RConn1\",\"RConn2\"],\"side\":\"RIGHT\"},\"type\":\"ConnectorPlacement.EquallySpacedRectSide\",\"uuid\":\"b280b04f-a99a-4e6d-85c5-70766288d403\"},{\"content\":{\"connectorIds\":[\"LConn1\"],\"side\":\"TOP\"},\"type\":\"ConnectorPlacement.EquallySpacedRectSide\",\"uuid\":\"c08bcee5-d382-416b-973d-9a8915fb752a\"},{\"content\":{\"connectorIds\":[\"RConn3\"],\"side\":\"BOTTOM\"},\"type\":\"ConnectorPlacement.EquallySpacedRectSide\",\"uuid\":\"7b01a887-c5d2-42f0-ba08-9cc04bc53540\"}]},\"type\":\"ConnectorPlacement.EquallySpacedConnector\",\"uuid\":\"7a443456-32e2-4b79-b23a-7f1f6189d6a8\"}],\"packageUris\":[\"http://schema.mathworks.com/mf0/Connector/R2020b\"],\"version\":\"1.0\"}"
  Subsystem7 : Subsystem
      settings: PortSchema="{\"entries\":[{\"content\":{\"sides\":[{\"content\":{\"connectorIds\":[\"In1\"]},\"type\":\"ConnectorPlacement.EquallySpacedRectSide\",\"uuid\":\"c40d362d-5d22-4f8a-8be9-1546116d818f\"},{\"content\":{\"connectorIds\":[\"RConn1\",\"RConn2\"],\"side\":\"RIGHT\"},\"type\":\"ConnectorPlacement.EquallySpacedRectSide\",\"uuid\":\"b280b04f-a99a-4e6d-85c5-70766288d403\"},{\"content\":{\"connectorIds\":[\"LConn1\"],\"side\":\"TOP\"},\"type\":\"ConnectorPlacement.EquallySpacedRectSide\",\"uuid\":\"c08bcee5-d382-416b-973d-9a8915fb752a\"},{\"content\":{\"connectorIds\":[\"RConn3\"],\"side\":\"BOTTOM\"},\"type\":\"ConnectorPlacement.EquallySpacedRectSide\",\"uuid\":\"7b01a887-c5d2-42f0-ba08-9cc04bc53540\"}]},\"type\":\"ConnectorPlacement.EquallySpacedConnector\",\"uuid\":\"7a443456-32e2-4b79-b23a-7f1f6189d6a8\"}],\"packageUris\":[\"http://schema.mathworks.com/mf0/Connector/R2020b\"],\"version\":\"1.0\"}"
  Subsystem8 : Subsystem
      settings: PortSchema="{\"entries\":[{\"content\":{\"sides\":[{\"content\":{\"connectorIds\":[\"In1\"]},\"type\":\"ConnectorPlacement.EquallySpacedRectSide\",\"uuid\":\"c40d362d-5d22-4f8a-8be9-1546116d818f\"},{\"content\":{\"connectorIds\":[\"RConn1\",\"RConn2\"],\"side\":\"RIGHT\"},\"type\":\"ConnectorPlacement.EquallySpacedRectSide\",\"uuid\":\"b280b04f-a99a-4e6d-85c5-70766288d403\"},{\"content\":{\"connectorIds\":[\"LConn1\"],\"side\":\"TOP\"},\"type\":\"ConnectorPlacement.EquallySpacedRectSide\",\"uuid\":\"c08bcee5-d382-416b-973d-9a8915fb752a\"},{\"content\":{\"connectorIds\":[\"RConn3\"],\"side\":\"BOTTOM\"},\"type\":\"ConnectorPlacement.EquallySpacedRectSide\",\"uuid\":\"7b01a887-c5d2-42f0-ba08-9cc04bc53540\"}]},\"type\":\"ConnectorPlacement.EquallySpacedConnector\",\"uuid\":\"7a443456-32e2-4b79-b23a-7f1f6189d6a8\"}],\"packageUris\":[\"http://schema.mathworks.com/mf0/Connector/R2020b\"],\"version\":\"1.0\"}"
  Subsystem9 : Subsystem
      settings: PortSchema="{\"entries\":[{\"content\":{\"sides\":[{\"content\":{\"connectorIds\":[\"In1\"]},\"type\":\"ConnectorPlacement.EquallySpacedRectSide\",\"uuid\":\"c40d362d-5d22-4f8a-8be9-1546116d818f\"},{\"content\":{\"connectorIds\":[\"RConn1\",\"RConn2\"],\"side\":\"RIGHT\"},\"type\":\"ConnectorPlacement.EquallySpacedRectSide\",\"uuid\":\"b280b04f-a99a-4e6d-85c5-70766288d403\"},{\"content\":{\"connectorIds\":[\"LConn1\"],\"side\":\"TOP\"},\"type\":\"ConnectorPlacement.EquallySpacedRectSide\",\"uuid\":\"c08bcee5-d382-416b-973d-9a8915fb752a\"},{\"content\":{\"connectorIds\":[\"RConn3\"],\"side\":\"BOTTOM\"},\"type\":\"ConnectorPlacement.EquallySpacedRectSide\",\"uuid\":\"7b01a887-c5d2-42f0-ba08-9cc04bc53540\"}]},\"type\":\"ConnectorPlacement.EquallySpacedConnector\",\"uuid\":\"7a443456-32e2-4b79-b23a-7f1f6189d6a8\"}],\"packageUris\":[\"http://schema.mathworks.com/mf0/Connector/R2020b\"],\"version\":\"1.0\"}"
  + : PMIOPort  Side=Left
  - : PMIOPort  Port=2  Side=Right
  SoC : Outport
  wires:
  Temp/1 -> Subsystem1/1(Temp), Subsystem2/1(Temp), Subsystem3/1(Temp), Subsystem4/1(Temp), Subsystem7/1(Temp), Subsystem9/1(Temp), Subsystem8/1(Temp), Subsystem6/1(Temp), Subsystem5/1(Temp), Subsystem/1(Temp)
  PS-Simulink Converter/1 -> SoC/1
  connections:
  Subsystem7/RConn1 -- PS Terminator11/LConn1
  Subsystem1/RConn1 -- PS Terminator17/LConn1
  Subsystem5/RConn2 -- PS Terminator5/LConn1
  Subsystem4/RConn1 -- PS Terminator14/LConn1
  Subsystem8/RConn2 -- PS Terminator8/LConn1
  Subsystem4/RConn2 -- PS Terminator4/LConn1
  Subsystem9/RConn1 -- PS-Simulink Converter/LConn1
  Subsystem5/RConn1 -- PS Terminator13/LConn1
  Subsystem6/RConn1 -- PS Terminator12/LConn1
  Subsystem/RConn1 -- PS Terminator18/LConn1
  Subsystem3/RConn2 -- PS Terminator3/LConn1
  Subsystem5/LConn1 -- Subsystem6/RConn3
  +/RConn1 -- Subsystem9/LConn1
  Subsystem6/RConn2 -- PS Terminator6/LConn1
  Subsystem2/RConn2 -- PS Terminator2/LConn1
  Subsystem9/RConn3 -- Subsystem8/LConn1
  Subsystem2/LConn1 -- Subsystem3/RConn3
  Subsystem/RConn2 -- PS Terminator/LConn1
  Subsystem7/LConn1 -- Subsystem8/RConn3
  Subsystem9/RConn2 -- PS Terminator9/LConn1
  Subsystem7/RConn2 -- PS Terminator7/LConn1
  Subsystem/LConn1 -- Subsystem1/RConn3
  Subsystem1/LConn1 -- Subsystem2/RConn3
  Subsystem/RConn3 -- -/RConn1
  Subsystem4/LConn1 -- Subsystem5/RConn3
  Subsystem6/LConn1 -- Subsystem7/RConn3
  Subsystem2/RConn1 -- PS Terminator16/LConn1
  Subsystem3/LConn1 -- Subsystem4/RConn3
  Subsystem3/RConn1 -- PS Terminator15/LConn1
  PS Terminator1/LConn1 -- Subsystem1/RConn2
  Subsystem8/RConn1 -- PS Terminator10/LConn1

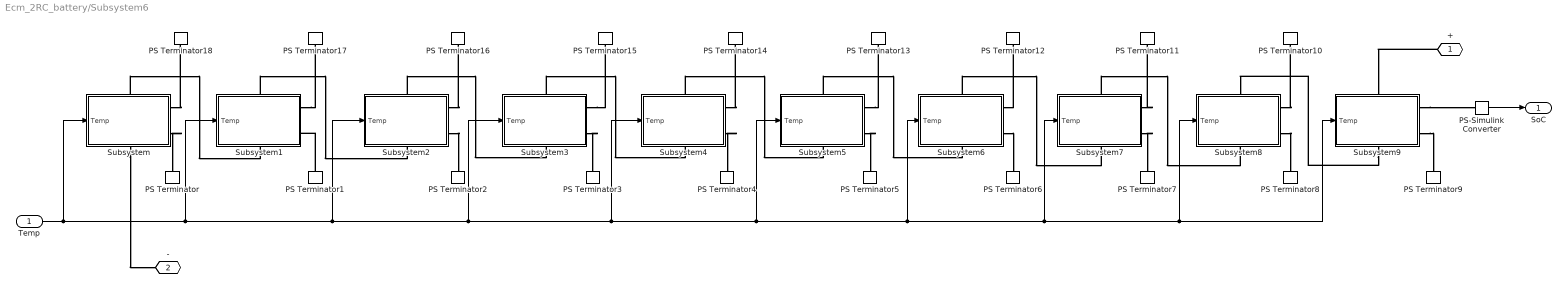
== system Ecm_2RC_battery/Subsystem6 ==
  Temp : Inport
  PS Terminator{,1..18} (19 alike) : fl_lib/Physical Signals/Sinks/PS Terminator
      settings: SourceProductBaseCode=PW,SS,VE
  PS-Simulink Converter : nesl_utility/PS-Simulink Converter  PhysicalDomain=network_engine_domain  SubClassName=ps_output  LeftPortType=input  RightPortType=output  PseudoPeriodic=off  Frequencies=[]  VectorFormat=inherit  Unit=inherit  AffineConversion=off
      settings: SourceProductBaseCode=SS,PW,VE
  Subsystem : Subsystem
      settings: PortSchema="{\"entries\":[{\"content\":{\"sides\":[{\"content\":{\"connectorIds\":[\"In1\"]},\"type\":\"ConnectorPlacement.EquallySpacedRectSide\",\"uuid\":\"c40d362d-5d22-4f8a-8be9-1546116d818f\"},{\"content\":{\"connectorIds\":[\"RConn1\",\"RConn2\"],\"side\":\"RIGHT\"},\"type\":\"ConnectorPlacement.EquallySpacedRectSide\",\"uuid\":\"b280b04f-a99a-4e6d-85c5-70766288d403\"},{\"content\":{\"connectorIds\":[\"LConn1\"],\"side\":\"TOP\"},\"type\":\"ConnectorPlacement.EquallySpacedRectSide\",\"uuid\":\"c08bcee5-d382-416b-973d-9a8915fb752a\"},{\"content\":{\"connectorIds\":[\"RConn3\"],\"side\":\"BOTTOM\"},\"type\":\"ConnectorPlacement.EquallySpacedRectSide\",\"uuid\":\"7b01a887-c5d2-42f0-ba08-9cc04bc53540\"}]},\"type\":\"ConnectorPlacement.EquallySpacedConnector\",\"uuid\":\"7a443456-32e2-4b79-b23a-7f1f6189d6a8\"}],\"packageUris\":[\"http://schema.mathworks.com/mf0/Connector/R2020b\"],\"version\":\"1.0\"}"
  Subsystem1 : Subsystem
      settings: PortSchema="{\"entries\":[{\"content\":{\"sides\":[{\"content\":{\"connectorIds\":[\"In1\"]},\"type\":\"ConnectorPlacement.EquallySpacedRectSide\",\"uuid\":\"c40d362d-5d22-4f8a-8be9-1546116d818f\"},{\"content\":{\"connectorIds\":[\"RConn1\",\"RConn2\"],\"side\":\"RIGHT\"},\"type\":\"ConnectorPlacement.EquallySpacedRectSide\",\"uuid\":\"b280b04f-a99a-4e6d-85c5-70766288d403\"},{\"content\":{\"connectorIds\":[\"LConn1\"],\"side\":\"TOP\"},\"type\":\"ConnectorPlacement.EquallySpacedRectSide\",\"uuid\":\"c08bcee5-d382-416b-973d-9a8915fb752a\"},{\"content\":{\"connectorIds\":[\"RConn3\"],\"side\":\"BOTTOM\"},\"type\":\"ConnectorPlacement.EquallySpacedRectSide\",\"uuid\":\"7b01a887-c5d2-42f0-ba08-9cc04bc53540\"}]},\"type\":\"ConnectorPlacement.EquallySpacedConnector\",\"uuid\":\"7a443456-32e2-4b79-b23a-7f1f6189d6a8\"}],\"packageUris\":[\"http://schema.mathworks.com/mf0/Connector/R2020b\"],\"version\":\"1.0\"}"
  Subsystem2 : Subsystem
      settings: PortSchema="{\"entries\":[{\"content\":{\"sides\":[{\"content\":{\"connectorIds\":[\"In1\"]},\"type\":\"ConnectorPlacement.EquallySpacedRectSide\",\"uuid\":\"c40d362d-5d22-4f8a-8be9-1546116d818f\"},{\"content\":{\"connectorIds\":[\"RConn1\",\"RConn2\"],\"side\":\"RIGHT\"},\"type\":\"ConnectorPlacement.EquallySpacedRectSide\",\"uuid\":\"b280b04f-a99a-4e6d-85c5-70766288d403\"},{\"content\":{\"connectorIds\":[\"LConn1\"],\"side\":\"TOP\"},\"type\":\"ConnectorPlacement.EquallySpacedRectSide\",\"uuid\":\"c08bcee5-d382-416b-973d-9a8915fb752a\"},{\"content\":{\"connectorIds\":[\"RConn3\"],\"side\":\"BOTTOM\"},\"type\":\"ConnectorPlacement.EquallySpacedRectSide\",\"uuid\":\"7b01a887-c5d2-42f0-ba08-9cc04bc53540\"}]},\"type\":\"ConnectorPlacement.EquallySpacedConnector\",\"uuid\":\"7a443456-32e2-4b79-b23a-7f1f6189d6a8\"}],\"packageUris\":[\"http://schema.mathworks.com/mf0/Connector/R2020b\"],\"version\":\"1.0\"}"
  Subsystem3 : Subsystem
      settings: PortSchema="{\"entries\":[{\"content\":{\"sides\":[{\"content\":{\"connectorIds\":[\"In1\"]},\"type\":\"ConnectorPlacement.EquallySpacedRectSide\",\"uuid\":\"c40d362d-5d22-4f8a-8be9-1546116d818f\"},{\"content\":{\"connectorIds\":[\"RConn1\",\"RConn2\"],\"side\":\"RIGHT\"},\"type\":\"ConnectorPlacement.EquallySpacedRectSide\",\"uuid\":\"b280b04f-a99a-4e6d-85c5-70766288d403\"},{\"content\":{\"connectorIds\":[\"LConn1\"],\"side\":\"TOP\"},\"type\":\"ConnectorPlacement.EquallySpacedRectSide\",\"uuid\":\"c08bcee5-d382-416b-973d-9a8915fb752a\"},{\"content\":{\"connectorIds\":[\"RConn3\"],\"side\":\"BOTTOM\"},\"type\":\"ConnectorPlacement.EquallySpacedRectSide\",\"uuid\":\"7b01a887-c5d2-42f0-ba08-9cc04bc53540\"}]},\"type\":\"ConnectorPlacement.EquallySpacedConnector\",\"uuid\":\"7a443456-32e2-4b79-b23a-7f1f6189d6a8\"}],\"packageUris\":[\"http://schema.mathworks.com/mf0/Connector/R2020b\"],\"version\":\"1.0\"}"
  Subsystem4 : Subsystem
      settings: PortSchema="{\"entries\":[{\"content\":{\"sides\":[{\"content\":{\"connectorIds\":[\"In1\"]},\"type\":\"ConnectorPlacement.EquallySpacedRectSide\",\"uuid\":\"c40d362d-5d22-4f8a-8be9-1546116d818f\"},{\"content\":{\"connectorIds\":[\"RConn1\",\"RConn2\"],\"side\":\"RIGHT\"},\"type\":\"ConnectorPlacement.EquallySpacedRectSide\",\"uuid\":\"b280b04f-a99a-4e6d-85c5-70766288d403\"},{\"content\":{\"connectorIds\":[\"LConn1\"],\"side\":\"TOP\"},\"type\":\"ConnectorPlacement.EquallySpacedRectSide\",\"uuid\":\"c08bcee5-d382-416b-973d-9a8915fb752a\"},{\"content\":{\"connectorIds\":[\"RConn3\"],\"side\":\"BOTTOM\"},\"type\":\"ConnectorPlacement.EquallySpacedRectSide\",\"uuid\":\"7b01a887-c5d2-42f0-ba08-9cc04bc53540\"}]},\"type\":\"ConnectorPlacement.EquallySpacedConnector\",\"uuid\":\"7a443456-32e2-4b79-b23a-7f1f6189d6a8\"}],\"packageUris\":[\"http://schema.mathworks.com/mf0/Connector/R2020b\"],\"version\":\"1.0\"}"
  Subsystem5 : Subsystem
      settings: PortSchema="{\"entries\":[{\"content\":{\"sides\":[{\"content\":{\"connectorIds\":[\"In1\"]},\"type\":\"ConnectorPlacement.EquallySpacedRectSide\",\"uuid\":\"c40d362d-5d22-4f8a-8be9-1546116d818f\"},{\"content\":{\"connectorIds\":[\"RConn1\",\"RConn2\"],\"side\":\"RIGHT\"},\"type\":\"ConnectorPlacement.EquallySpacedRectSide\",\"uuid\":\"b280b04f-a99a-4e6d-85c5-70766288d403\"},{\"content\":{\"connectorIds\":[\"LConn1\"],\"side\":\"TOP\"},\"type\":\"ConnectorPlacement.EquallySpacedRectSide\",\"uuid\":\"c08bcee5-d382-416b-973d-9a8915fb752a\"},{\"content\":{\"connectorIds\":[\"RConn3\"],\"side\":\"BOTTOM\"},\"type\":\"ConnectorPlacement.EquallySpacedRectSide\",\"uuid\":\"7b01a887-c5d2-42f0-ba08-9cc04bc53540\"}]},\"type\":\"ConnectorPlacement.EquallySpacedConnector\",\"uuid\":\"7a443456-32e2-4b79-b23a-7f1f6189d6a8\"}],\"packageUris\":[\"http://schema.mathworks.com/mf0/Connector/R2020b\"],\"version\":\"1.0\"}"
  Subsystem6 : Subsystem
      settings: PortSchema="{\"entries\":[{\"content\":{\"sides\":[{\"content\":{\"connectorIds\":[\"In1\"]},\"type\":\"ConnectorPlacement.EquallySpacedRectSide\",\"uuid\":\"c40d362d-5d22-4f8a-8be9-1546116d818f\"},{\"content\":{\"connectorIds\":[\"RConn1\",\"RConn2\"],\"side\":\"RIGHT\"},\"type\":\"ConnectorPlacement.EquallySpacedRectSide\",\"uuid\":\"b280b04f-a99a-4e6d-85c5-70766288d403\"},{\"content\":{\"connectorIds\":[\"LConn1\"],\"side\":\"TOP\"},\"type\":\"ConnectorPlacement.EquallySpacedRectSide\",\"uuid\":\"c08bcee5-d382-416b-973d-9a8915fb752a\"},{\"content\":{\"connectorIds\":[\"RConn3\"],\"side\":\"BOTTOM\"},\"type\":\"ConnectorPlacement.EquallySpacedRectSide\",\"uuid\":\"7b01a887-c5d2-42f0-ba08-9cc04bc53540\"}]},\"type\":\"ConnectorPlacement.EquallySpacedConnector\",\"uuid\":\"7a443456-32e2-4b79-b23a-7f1f6189d6a8\"}],\"packageUris\":[\"http://schema.mathworks.com/mf0/Connector/R2020b\"],\"version\":\"1.0\"}"
  Subsystem7 : Subsystem
      settings: PortSchema="{\"entries\":[{\"content\":{\"sides\":[{\"content\":{\"connectorIds\":[\"In1\"]},\"type\":\"ConnectorPlacement.EquallySpacedRectSide\",\"uuid\":\"c40d362d-5d22-4f8a-8be9-1546116d818f\"},{\"content\":{\"connectorIds\":[\"RConn1\",\"RConn2\"],\"side\":\"RIGHT\"},\"type\":\"ConnectorPlacement.EquallySpacedRectSide\",\"uuid\":\"b280b04f-a99a-4e6d-85c5-70766288d403\"},{\"content\":{\"connectorIds\":[\"LConn1\"],\"side\":\"TOP\"},\"type\":\"ConnectorPlacement.EquallySpacedRectSide\",\"uuid\":\"c08bcee5-d382-416b-973d-9a8915fb752a\"},{\"content\":{\"connectorIds\":[\"RConn3\"],\"side\":\"BOTTOM\"},\"type\":\"ConnectorPlacement.EquallySpacedRectSide\",\"uuid\":\"7b01a887-c5d2-42f0-ba08-9cc04bc53540\"}]},\"type\":\"ConnectorPlacement.EquallySpacedConnector\",\"uuid\":\"7a443456-32e2-4b79-b23a-7f1f6189d6a8\"}],\"packageUris\":[\"http://schema.mathworks.com/mf0/Connector/R2020b\"],\"version\":\"1.0\"}"
  Subsystem8 : Subsystem
      settings: PortSchema="{\"entries\":[{\"content\":{\"sides\":[{\"content\":{\"connectorIds\":[\"In1\"]},\"type\":\"ConnectorPlacement.EquallySpacedRectSide\",\"uuid\":\"c40d362d-5d22-4f8a-8be9-1546116d818f\"},{\"content\":{\"connectorIds\":[\"RConn1\",\"RConn2\"],\"side\":\"RIGHT\"},\"type\":\"ConnectorPlacement.EquallySpacedRectSide\",\"uuid\":\"b280b04f-a99a-4e6d-85c5-70766288d403\"},{\"content\":{\"connectorIds\":[\"LConn1\"],\"side\":\"TOP\"},\"type\":\"ConnectorPlacement.EquallySpacedRectSide\",\"uuid\":\"c08bcee5-d382-416b-973d-9a8915fb752a\"},{\"content\":{\"connectorIds\":[\"RConn3\"],\"side\":\"BOTTOM\"},\"type\":\"ConnectorPlacement.EquallySpacedRectSide\",\"uuid\":\"7b01a887-c5d2-42f0-ba08-9cc04bc53540\"}]},\"type\":\"ConnectorPlacement.EquallySpacedConnector\",\"uuid\":\"7a443456-32e2-4b79-b23a-7f1f6189d6a8\"}],\"packageUris\":[\"http://schema.mathworks.com/mf0/Connector/R2020b\"],\"version\":\"1.0\"}"
  Subsystem9 : Subsystem
      settings: PortSchema="{\"entries\":[{\"content\":{\"sides\":[{\"content\":{\"connectorIds\":[\"In1\"]},\"type\":\"ConnectorPlacement.EquallySpacedRectSide\",\"uuid\":\"c40d362d-5d22-4f8a-8be9-1546116d818f\"},{\"content\":{\"connectorIds\":[\"RConn1\",\"RConn2\"],\"side\":\"RIGHT\"},\"type\":\"ConnectorPlacement.EquallySpacedRectSide\",\"uuid\":\"b280b04f-a99a-4e6d-85c5-70766288d403\"},{\"content\":{\"connectorIds\":[\"LConn1\"],\"side\":\"TOP\"},\"type\":\"ConnectorPlacement.EquallySpacedRectSide\",\"uuid\":\"c08bcee5-d382-416b-973d-9a8915fb752a\"},{\"content\":{\"connectorIds\":[\"RConn3\"],\"side\":\"BOTTOM\"},\"type\":\"ConnectorPlacement.EquallySpacedRectSide\",\"uuid\":\"7b01a887-c5d2-42f0-ba08-9cc04bc53540\"}]},\"type\":\"ConnectorPlacement.EquallySpacedConnector\",\"uuid\":\"7a443456-32e2-4b79-b23a-7f1f6189d6a8\"}],\"packageUris\":[\"http://schema.mathworks.com/mf0/Connector/R2020b\"],\"version\":\"1.0\"}"
  + : PMIOPort  Side=Left
  - : PMIOPort  Port=2  Side=Right
  SoC : Outport
  wires:
  Temp/1 -> Subsystem1/1(Temp), Subsystem2/1(Temp), Subsystem3/1(Temp), Subsystem4/1(Temp), Subsystem7/1(Temp), Subsystem9/1(Temp), Subsystem8/1(Temp), Subsystem6/1(Temp), Subsystem5/1(Temp), Subsystem/1(Temp)
  PS-Simulink Converter/1 -> SoC/1
  connections:
  Subsystem7/RConn1 -- PS Terminator11/LConn1
  Subsystem1/RConn1 -- PS Terminator17/LConn1
  Subsystem5/RConn2 -- PS Terminator5/LConn1
  Subsystem4/RConn1 -- PS Terminator14/LConn1
  Subsystem8/RConn2 -- PS Terminator8/LConn1
  Subsystem4/RConn2 -- PS Terminator4/LConn1
  Subsystem9/RConn1 -- PS-Simulink Converter/LConn1
  Subsystem5/RConn1 -- PS Terminator13/LConn1
  Subsystem6/RConn1 -- PS Terminator12/LConn1
  Subsystem/RConn1 -- PS Terminator18/LConn1
  Subsystem3/RConn2 -- PS Terminator3/LConn1
  Subsystem5/LConn1 -- Subsystem6/RConn3
  +/RConn1 -- Subsystem9/LConn1
  Subsystem6/RConn2 -- PS Terminator6/LConn1
  Subsystem2/RConn2 -- PS Terminator2/LConn1
  Subsystem9/RConn3 -- Subsystem8/LConn1
  Subsystem2/LConn1 -- Subsystem3/RConn3
  Subsystem/RConn2 -- PS Terminator/LConn1
  Subsystem7/LConn1 -- Subsystem8/RConn3
  Subsystem9/RConn2 -- PS Terminator9/LConn1
  Subsystem7/RConn2 -- PS Terminator7/LConn1
  Subsystem/LConn1 -- Subsystem1/RConn3
  Subsystem1/LConn1 -- Subsystem2/RConn3
  Subsystem/RConn3 -- -/RConn1
  Subsystem4/LConn1 -- Subsystem5/RConn3
  Subsystem6/LConn1 -- Subsystem7/RConn3
  Subsystem2/RConn1 -- PS Terminator16/LConn1
  Subsystem3/LConn1 -- Subsystem4/RConn3
  Subsystem3/RConn1 -- PS Terminator15/LConn1
  PS Terminator1/LConn1 -- Subsystem1/RConn2
  Subsystem8/RConn1 -- PS Terminator10/LConn1
